simulink model "mVeh_fun_tbm"  (R2023b)
settings: Solver=FixedStepDiscrete  StartTime=0.0  StopTime=Parm_cnv_simulink_stopTime  FixedStep=Const_cnv_fundmt_stepSize  RelTol=1e-3  EnableMultiTasking=on
InitFcn:
  | preLoadFun
undefined symbols (not defined in the file or in its folder): Calib_pirelle_presSnr_x8, Calib_roadTriger_x6, Calib_tbm_brkBts_x8, Calib_tbm_ctr_x8, Calib_tbm_sensor_x4, Calib_tbm_strDistb_x8, Calib_tbm_supCtr_x8, CtrSet_tbm_enab_x8, IO397, Parm_tbmVeh_sig_max_numInvalid, Parm_tbmVeh_sig_tolerate_numInvalid
libraries: canmsglib x34, speedgoatlib_IO691 x19, MyLibrary x5, libtb_gen_canMsgCntr x5, speedgoatlib_fpga_analog_io x1, simulink x1, speedgoatlib_fpga x1, lib_decmp_CtrSet_tbm_enab_x8 x1, lib_decmp_Calib_tbm_brkPreTriger_x6 x1, lib_decmp_Calib_tbm_sensor_x4 x1
(part 1 of 3)
Description:
  | - Add preLoadFun.m into Callbacks InitFcn
  | - Combine Sensata and Pirelle sensor inputs into one subsystem
  | - Two enumerators: defEnum_fun_tbm.m && def_vehFun_Enum.m
settings Model: SimulationMode=external  PauseTimes=49.73  NumberOfSteps=20  PacingRate=112  Creator=jianjun.gao  LastModifiedBy=nolalala
settings SolverCC: ConcurrentTasks=on  AlgebraicLoopSolver=LineSearch  AutoInsertRateTranBlk=on
settings DataIOCC: LimitDataPoints=on  SaveFormat=StructureWithTime  ReturnWorkspaceOutputs=off
settings OptimizationCC: BlockReduction=off  DefaultUnderspecifiedDataType=single  OptimizeBlockIOStorage=off  EnhancedBackFolding=on  PassReuseOutputArgsThreshold=0  ExpressionDepthLimit=2147483647  OptimizeBlockOrder=speed  DifferentSizesBufferReuse=on
settings DebuggingCC: UnderspecifiedInitializationDetection=Classic  MergeDetectMultiDrivingBlocksExec=none  SolverPrmCheckMsg=warning  ParameterTunabilityLossMsg=error  FcnCallInpInsideContextMsg=warning  UnconnectedInputMsg=warning  UnconnectedOutputMsg=warning  UnconnectedLineMsg=warning  BusObjectLabelMismatch=error  AllowSymbolicDim=off  StateNameClashWarn=warning  SFUnexpectedBacktrackingDiag=warning  SFNoUnconditionalDefaultTransitionDiag=warning  SFExecutionAtInitializationDiag=none  ArithmeticOperatorsInVariantConditions=warning
settings HardwareCC: ProdBitPerPointer=32  ProdBitPerSizeT=32  ProdBitPerPtrDiffT=32  ProdLargestAtomicFloat=None  ProdWordSize=32  ProdLongLongMode=on  ProdHWDeviceType=Generic->32-bit x86 compatible
settings ModelReferenceCC: EnableRefExpFcnMdlSchedulingChecks=on  PropagateSignalLabelsOutOfModel=off
settings SFSimCC: SimUseLocalCustomCode=off  MATLABDynamicMemAlloc=off  CustomCodeUndefinedFunction=UseInterfaceOnly
settings RTWCC: Description=Simulink Real-Time  SystemTargetFile=slrt.tlc  PackageName=addn_compled  TemplateMakefile=slrt_default_tmf  RTWUseLocalCustomCode=off  RTWUseSimCustomCode=on  BuildConfiguration=Faster Runs  CodeExecutionProfiling=on  RTWCompilerOptimization=on
settings CodeAppCC: ForceParamTrailComments=on  MaxIdLength=63  OperatorAnnotations=on
settings SimulinkRealTimeCC: SupportVariableSizeSignals=on  OptimizeReductions=off  RL32LogTETModifier=off  xPCConcurrentTasks=on
settings ConfigComp: CovMetricSettings=dw  CovSaveCumulativeToWorkspaceVar=on  CovSaveSingleToWorkspaceVar=on  CovExternalEMLEnable=off
settings SimscapeCC: SimscapeNormalizeSystem=off
settings ConfigurationSet: Description=SimMechanics 2G

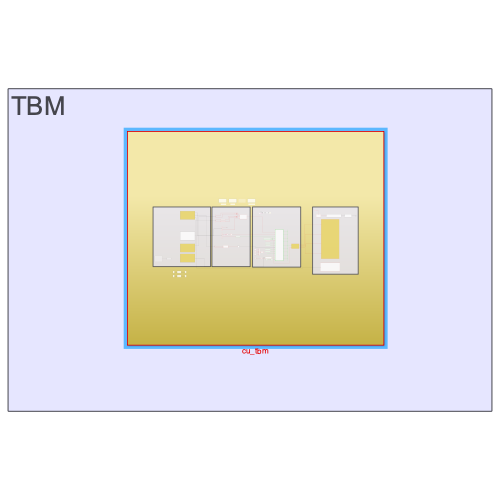
[thumbnail: Simulink's stored preview of the top-level diagram]
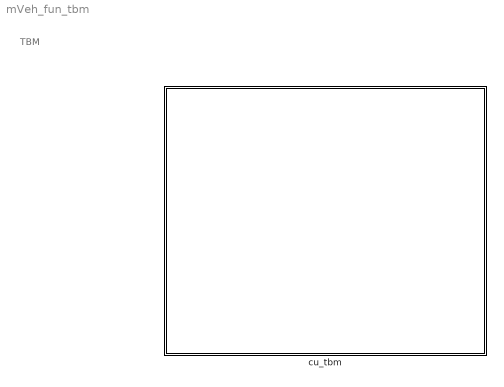
== system mVeh_fun_tbm ==
  note: TBM
  cu_tbm : Subsystem

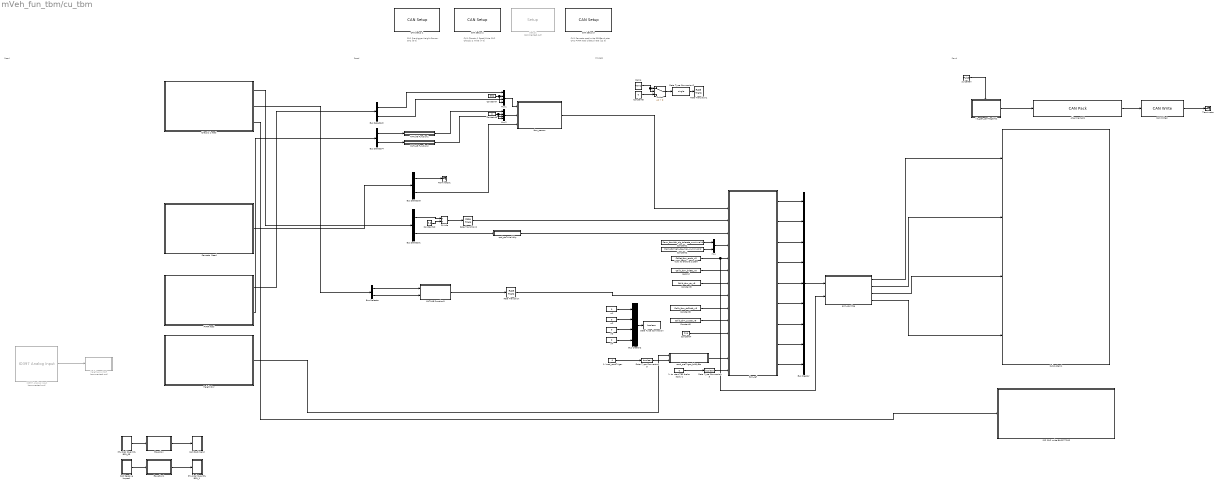
== system mVeh_fun_tbm/cu_tbm ==
  note: CH1 Pre-trigger Height Sensor
      | CH2
      | [6 0]
  note: Send
  note: Process
  note: Read
  note: CH1 Chassis 1 Read/Write
      | CH2 Chassis 2 Write
      | [7 0]
  note: CH1 Sensata read/write 500Baud rate
      | CH2 PVRR read 1kBaud rate
      | [12 0]
  note: Read
  1: load_roadTriger : Constant  Value=0  OutDataTypeStr=uint8  SampleTime=-1
  1: to  start TBS brake apply1 : Constant  Value=0  OutDataTypeStr=uint8  SampleTime=-1
  Alignment_01 : canmsglib/CAN Pack  CANdbFile=C:\Users\bowen.zheng\Desktop\spdGoat_prj_20230526_mod\spdGoat_prj_20230526\support\dbc\TBM_mix.dbc  MsgList=Alignment_01  MsgName=Alignment_01  MsgIDType=Standard (11-bit identifier)  MsgIdentifier=1043  MsgLength=2  Remote=off  ApplyMinMax=off  BusOutput=off  SignalInfo={'Alignment_TimeStamp','8','16','BE','unsigned','Standard','0','1','0','0','65535'}
      settings: DataFormat=CANdb specified signals
  Bus Creator : BusCreator  Inputs=9
  Bus Creator2 : BusCreator  Inputs=4
  Bus Selector : BusSelector  OutputSignals=BCU_04_BrkPedlTrvlCalSts,BCU_04_BrkPedlSts
  Bus Selector1 : BusSelector  OutputSignals=BCU_04_VehSpd,BCU_04_VehSpdSts
  Bus Selector2 : BusSelector  OutputSignals=PVRR_press_front,PVRR_press_rear
  Bus Selector3 : BusSelector  OutputSignals=Sensata_burst_pressure,Sensata_burst_flag
  Bus Selector4 : BusSelector  OutputSignals=PVRR_timestamp_front,PVRR_timestamp_rear
  CAN Pack Send : Subsystem
  CAN Receive Unpack : Subsystem
  CAN Setup 1 : speedgoatlib_IO691/CAN Setup   moduletype=IO691  id=1  pciSlot=[6 0]  chn1=CAN (HS)  chn2=CAN (HS)  chn3=Disabled  chn4=Disabled  initStruct=[]  termStruct=[]  ArbitrationbdrChn1=500 kBaud  ArbitrationManbdrChn1=[2,16,63,16]  FdbdrChn1=5.0 MBaud  FdManbdrChn1=[2,2,5,2]  ArbitrationbdrChn2=500 kBaud  ArbitrationManbdrChn2=[2,16,63,16]  FdbdrChn2=5.0 MBaud  FdManbdrChn2=[2,2,5,2]  ArbitrationbdrChn3=1.0 MBaud  ArbitrationManbdrChn3=[2,8,31,8]  FdbdrChn3=5.0 MBaud  FdManbdrChn3=[2,2,5,2]  ArbitrationbdrChn4=1.0 MBaud  ArbitrationManbdrChn4=[2,8,31,8]  FdbdrChn4=5.0 MBaud  FdManbdrChn4=[2,2,5,2]  moduleInitValues=[691 1 6 0]
  CAN Setup 2 : speedgoatlib_IO691/CAN Setup   moduletype=IO691  id=2  pciSlot=[7 0]  chn1=CAN (HS)  chn2=CAN (HS)  chn3=Disabled  chn4=Disabled  initStruct=[]  termStruct=[]  ArbitrationbdrChn1=500 kBaud  ArbitrationManbdrChn1=[2,16,63,16]  FdbdrChn1=5.0 MBaud  FdManbdrChn1=[2,2,5,2]  ArbitrationbdrChn2=500 kBaud  ArbitrationManbdrChn2=[2,16,63,16]  FdbdrChn2=5.0 MBaud  FdManbdrChn2=[2,2,5,2]  ArbitrationbdrChn3=1.0 MBaud  ArbitrationManbdrChn3=[2,8,31,8]  FdbdrChn3=5.0 MBaud  FdManbdrChn3=[2,2,5,2]  ArbitrationbdrChn4=1.0 MBaud  ArbitrationManbdrChn4=[2,8,31,8]  FdbdrChn4=5.0 MBaud  FdManbdrChn4=[2,2,5,2]  moduleInitValues=[691 2 7 0]
  CAN Setup 3 : speedgoatlib_IO691/CAN Setup   moduletype=IO691  id=4  pciSlot=[12 0]  chn1=CAN (HS)  chn2=CAN (HS)  chn3=Disabled  chn4=Disabled  initStruct=[]  termStruct=[]  ArbitrationbdrChn1=500 kBaud  ArbitrationManbdrChn1=[2,16,63,16]  FdbdrChn1=5.0 MBaud  FdManbdrChn1=[2,2,5,2]  ArbitrationbdrChn2=1.0 MBaud  ArbitrationManbdrChn2=[2,8,31,8]  FdbdrChn2=5.0 MBaud  FdManbdrChn2=[2,2,5,2]  ArbitrationbdrChn3=1.0 MBaud  ArbitrationManbdrChn3=[2,8,31,8]  FdbdrChn3=5.0 MBaud  FdManbdrChn3=[2,2,5,2]  ArbitrationbdrChn4=1.0 MBaud  ArbitrationManbdrChn4=[2,8,31,8]  FdbdrChn4=5.0 MBaud  FdManbdrChn4=[2,2,5,2]  moduleInitValues=[691 4 12 0]
  CAN Write2 : speedgoatlib_IO691/CAN Write  id=4  ts=0.01  channel=1  messageType=CAN  enableStatusPort=on  canType=CAN (HS)  initValues=[691 4 0.01 0 1 1 1]
  Chassis 1 read : Subsystem
  Constant1 : Constant  Value=Parm_tbmVeh_sig_tolerate_numInvalid  OutDataTypeStr=int8  SampleTime=-1
  Constant10 : Constant  Value=3.6  OutDataTypeStr=single
  Constant2 : Constant  Value=Parm_tbmVeh_sig_max_numInvalid  OutDataTypeStr=int8  SampleTime=-1
  Constant3 : Constant  Value=Calib_tbm_supCtr_x8  OutDataTypeStr=single  SampleTime=-1
  Constant4 : Constant  Value=true  OutDataTypeStr=boolean  SampleTime=-1
  Constant5 : Constant  Value=Calib_tbm_ctr_x8  OutDataTypeStr=single  SampleTime=-1
  Constant6 : Constant  Value=0  OutDataTypeStr=single
  Constant7 : Constant  Value=350  OutDataTypeStr=single  SampleTime=-1
  Constant8 : Constant  Value=Calib_tbm_strDistb_x8  OutDataTypeStr=single  SampleTime=-1
  Constant9 : Constant  Value=0  OutDataTypeStr=single  SampleTime=-1
  Data Type Conversion : DataTypeConversion  OutDataTypeStr=boolean  SaturateOnIntegerOverflow=off  RndMeth=Floor
  Data Type Conversion2 : DataTypeConversion  OutDataTypeStr=single  SaturateOnIntegerOverflow=off  RndMeth=Floor
  Data Type Conversion3 : DataTypeConversion  OutDataTypeStr=boolean  RndMeth=Nearest  SaturateOnIntegerOverflow=off
  Data Type Conversion5 : DataTypeConversion  OutDataTypeStr=boolean  RndMeth=Nearest  SaturateOnIntegerOverflow=off
  Divide : Product  Inputs=*/  OutDataTypeStr=single  RndMeth=Nearest
  Equation : Subsystem
  Equation1 : Subsystem
  Height Snr : Subsystem
  ID2 CH2 write BAICC TPMS : Subsystem
  IO397 Analog Input : speedgoatlib_fpga_analog_io/IO397 Analog Input  Commented=on  id=3  chan=[2:2]  range=+-10 V  trigger=Initiator  ts=0.001  pciSlot=-1  board=Please select...
  MATLAB Function1 : MATLAB Function  TreatAsAtomicUnit=on
  MATLAB Function2 : MATLAB Function  TreatAsAtomicUnit=on
  MATLAB Function3 : MATLAB Function  TreatAsAtomicUnit=on
  Mux : Mux  Inputs=2
  Mux1 : Mux
  Mux2 : Mux
  PVRR read : Subsystem
  Physical Quantity BCU_05 : Subsystem
  Physical Quantity BCU_1 : Subsystem
  Ramp : simulink/Sources/Ramp  slope=-2  start=10  InitialOutput=100
  Rate Transition : RateTransition
  Rate Transition1 : RateTransition
  Rate Transition2 : RateTransition
  Sensata  Read : Subsystem
  Setup1 : speedgoatlib_fpga/Setup/Setup  Commented=on  board=IO397-50k  id=3  device_id=1  frontIO=None  rearIO=None  bitstreamFile=speedgoat_IO397_50k_all_io.mat  rev=2.1  timestamp_string=06/12/19 11:07:30  fpgaFreq=75 MHz  fpgaTick=13.33 ns  ProgSpiFlash=off  ProgBPIFlash=off  pciSlot=-1  PullRPort0=pull-up 3.3V  VioPort0=3.3V  PullRPort1=pull-up 3.3V  VioPort1=3.3V  PullRPort2=pull-up 3.3V  VioPort2=3.3V  PullRPort3=pull-up 3.3V  VioPort3=3.3V  PullRPort4=pull-up 3.3V  VioPort4=3.3V  PullRPort5=pull-up 3.3V  VioPort5=3.3V  PullRPort6=pull-up 3.3V  VioPort6=3.3V  PullRPort15=pull-up 3.3V  PullRPort31=pull-up 3.3V  PullRPort47=pull-up 3.3V  PullRPort63=pull-up 3.3V
  Subsystem1 : Subsystem
  Switch : Switch  Criteria=u2 > Threshold  SaturateOnIntegerOverflow=off  InputSameDT=off
  Terminator : Terminator
  Terminator1 : Terminator
  asm_canMsg : Subsystem
  height_snr_VtoH : MATLAB Function  Commented=on  TreatAsAtomicUnit=on
  lib_gen_canMsgCntr1 : Stateflow chart  AncestorBlock=libtb_gen_canMsgCntr/lib_gen_canMsgCntr  TreatAsAtomicUnit=on
  pulseGen : DiscretePulseGenerator  PulseType=Time based  Period=0.01  PulseWidth=50
  road_preTriger_brkByBts : Subsystem
  second : Constant  Value=Calib_tbm_brkBts_x8  OutDataTypeStr=single  SampleTime=-1
  spd_stsToValidity : MATLAB Function  TreatAsAtomicUnit=on
  tbm_ref : ModelReference  ModelNameDialog=tbm_ref.slx  SimulationMode=Normal  ModelReferenceVersion=1.941
  tbm_sensor : Subsystem
  true: to enable system : Constant  Value=CtrSet_tbm_enab_x8  OutDataTypeStr=boolean  SampleTime=-1
  w1 : Constant  Value=0  OutDataTypeStr=single
  "w2 " : Constant  Value=0  OutDataTypeStr=single  SampleTime=-1
  w3 : Constant  Value=0  OutDataTypeStr=single  SampleTime=-1
  w4 : Constant  Value=0  OutDataTypeStr=single  SampleTime=-1
  wires:
  Chassis 1 read/2(BCU_04_BrkPedl_w_Sts) -> Bus Selector/1
  Chassis 1 read/1(BCU_04_VehSpd_w_Validity) -> Bus Selector1/1
  Sensata  Read/1(TPMS_TireBurst) -> Bus Selector3/1
  Chassis 1 read/3(BGW_02_VehState) -> ID2 CH2 write BAICC TPMS/1(VehState)
  Bus Creator2/1 -> Data Type Conversion/1
  "w2 "/1 -> Bus Creator2/2
  w1/1 -> Bus Creator2/1
  Bus Creator/1 -> asm_canMsg/1(cu_tbm)
  tbm_ref/1 -> Bus Creator/1  "tbm_st"
  tbm_ref/3 -> Bus Creator/3  "btsSimuDrBrk_mcp"
  tbm_ref/5 -> Bus Creator/5  "tbmModfBrk_pTgt_4w"
  tbm_ref/8 -> Bus Creator/8  "susp_ctrActv_4w"
  tbm_ref/2 -> Bus Creator/2  "btsSimuDrBrk_actv"
  tbm_ref/4 -> Bus Creator/4  "tbmModfBrk_actv_4w"
  spd_stsToValidity/1(spd_valid) -> tbm_ref/4
  tbm_ref/6 -> Bus Creator/6  "str_distbCtr_actv"
  tbm_ref/9 -> Bus Creator/9  "susp_pTgt_4w"
  tbm_ref/7 -> Bus Creator/7  "str_distbCtr_angTgt"
  Bus Selector3/1 -> Terminator1/1  "<Sensata_burst_pressure>"
  Bus Selector1/2 -> spd_stsToValidity/1(spd_status)  "<BCU_04_VehSpdSts>"
  Bus Selector/1 -> MATLAB Function3/1(brkPdlTrvlCalSts)  "<BCU_04_BrkPedlTrvlCalSts>"
  Bus Selector/2 -> MATLAB Function3/2(brkPdlSts)  "<BCU_04_BrkPedlSts>"
  Ramp/1 -> Switch/2, Switch/1
  asm_canMsg/4(bus_to_ch2_VCU_14) -> Subsystem1/4(busTo_vcu_14)
  asm_canMsg/3(busTo_adc1_eps_02) -> Subsystem1/3(busTo_adc1_eps_02)
  asm_canMsg/2(busTo_adc1_eps_01) -> Subsystem1/2(busTo_adc1_eps_01)
  asm_canMsg/1(busTo_ch1_tbm_02) -> Subsystem1/1(busTo_ch1_tbm_02)
  Constant6/1 -> Switch/3
  Switch/1 -> Data Type Conversion2/1
  Data Type Conversion2/1 -> Rate Transition1/1
  Bus Selector3/2 -> tbm_sensor/3(sansata_boutFlag_4w)  "<Sensata_burst_flag>"
  w3/1 -> Bus Creator2/3
  w4/1 -> Bus Creator2/4
  Bus Selector1/1 -> Divide/1  "<BCU_04_VehSpd>"
  Constant10/1 -> Divide/2
  Rate Transition2/1 -> tbm_ref/3
  Divide/1 -> Rate Transition2/1
  PVRR read/1(PVRR_press) -> Bus Selector2/1
  PVRR read/2(PVRR_timestamp) -> Bus Selector4/1
  Bus Selector2/1 -> Mux1/1  "<PVRR_press_front>"
  Bus Selector2/2 -> Mux1/3  "<PVRR_press_rear>"
  Bus Selector4/1 -> MATLAB Function1/1(timestamp)  "<PVRR_timestamp_front>"
  Bus Selector4/2 -> MATLAB Function2/1(timestamp)  "<PVRR_timestamp_rear>"
  IO397 Analog Input/1 -> height_snr_VtoH/1(snr_volt)  "Analog Input"
  pulseGen/1 -> lib_gen_canMsgCntr1/Trigger
  Alignment_01/1 -> CAN Write2/1
  lib_gen_canMsgCntr1/1(count) -> Alignment_01/1  "Alightment_cout"
  CAN Write2/1 -> Terminator/1  "state"
  1: to  start TBS brake apply1/1 -> Data Type Conversion3/1  "handTriger"
  Data Type Conversion3/1 -> tbm_ref/15
  Data Type Conversion5/1 -> road_preTriger_brkByBts/2(load_roadTrigr)
  road_preTriger_brkByBts/1(road_trigred) -> tbm_ref/14  "road_trigred"
  1: load_roadTriger/1 -> Data Type Conversion5/1  "load_roadTriger"
  Constant4/1 -> tbm_ref/12
  Constant3/1 -> tbm_ref/11
  Constant8/1 -> tbm_ref/10
  MATLAB Function3/1(dr_isBrkg) -> Rate Transition/1  "dr_isBrkg"
  Constant5/1 -> tbm_ref/8
  second/1 -> tbm_ref/7
  true: to enable system/1 -> tbm_ref/6, asm_canMsg/2(CtrSet_tbm_enab_x8)
  Mux/1 -> tbm_ref/5
  Constant1/1 -> Mux/1
  Constant2/1 -> Mux/2
  Height Snr/1(Height Snr) -> road_preTriger_brkByBts/1(measured_tgrGap)  "height_snr"
  Rate Transition/1 -> tbm_ref/9
  Constant9/1 -> Mux2/4, Mux2/2
  Constant7/1 -> Mux1/2, Mux1/4
  Mux1/1 -> tbm_sensor/1(pirelle_tryPres_4w)
  Mux2/1 -> tbm_sensor/2(pirelle_snrTime_4w)
  tbm_sensor/1(snr_boutFlag_4w) -> tbm_ref/2  "snr_blouFlag_4w"
  MATLAB Function1/1(timestamp_sec) -> Mux2/1  "ts_sec_front"
  MATLAB Function2/1(timestamp_sec) -> Mux2/3  "ts_sec_rear"
  Physical Quantity BCU_05/1(BCU_05) -> Equation/1(BCU_05)
  Equation/1(Transformed) -> CAN Pack Send/1(Input)
  CAN Receive Unpack/1(Output) -> Equation1/1(ADC_Waypoint)
  Equation1/1(Transformed) -> Physical Quantity BCU_1/1(Input)

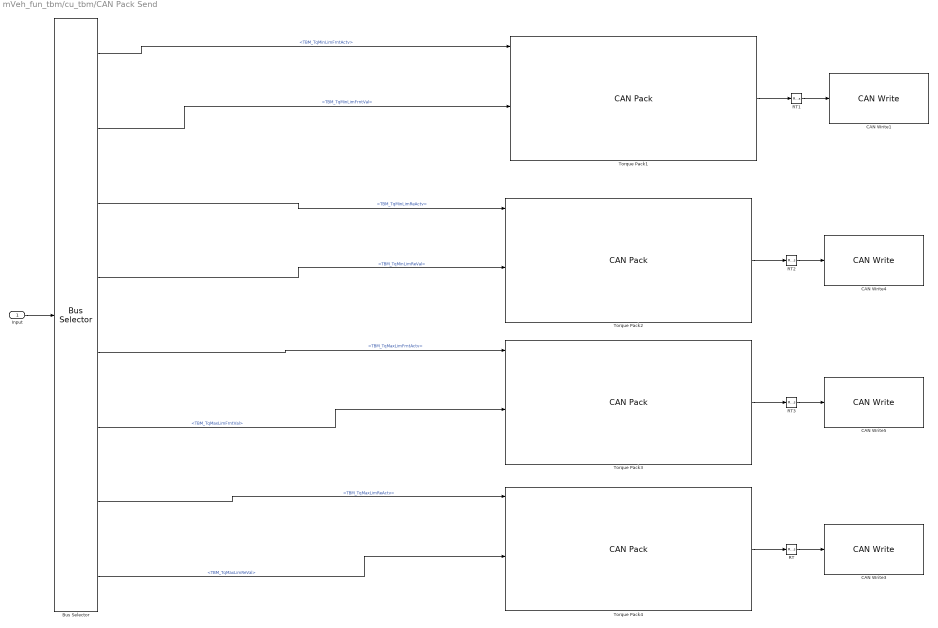
== system mVeh_fun_tbm/cu_tbm/CAN Pack Send ==
  Input : Inport
  Bus Selector : BusSelector  OutputSignals=TBM_TqMinLimFrntActv,TBM_TqMinLimFrntVal,TBM_TqMinLimReActv,TBM_TqMinLimReVal,TBM_TqMaxLimFrntActv,TBM_TqMaxLimFrntVal,TBM_TqMaxLimReActv,TBM_TqMaxLimReVal
  CAN Write{1,3..5} (4 alike) : speedgoatlib_IO691/CAN Write  id=2  ts=0.02  channel=1  messageType=CAN  enableStatusPort=off  canType=CAN (HS)  initValues=[691 2 0.02 0 1 1 0]
  RT{,1..3} (4 alike) : RateTransition  OutPortSampleTime=0.02
  Torque Pack1 : canmsglib/CAN Pack  CANdbFile=.\support\dbc\NIO_NT2_Chassis2_CAN_Official_Release_V_1_1_DA_02.dbc  MsgList=ADC1_WayPoint01  MsgName=ADC1_WayPoint01  MsgIDType=Standard (11-bit identifier)  MsgIdentifier=214  MsgLength=8  Remote=off  ApplyMinMax=off  BusOutput=off  SignalInfo={'LD_Confidence_1','24','4','BE','unsigned','Standard','0','0.1','0','0','1.5';'LD_First_End_1','51','7','BE','unsigned','Standard','0','1','0','0','127';'LD_First_Start_1','16','8','BE','unsigned','Standard','0','0.1','0','0','25.5';'LD_First_Type_1','28','4','BE','unsigned','Standard','0','1','0','0','15';'LD_Line_First_C0_1','56','11','BE','unsigned','Standard','0','0.01','-10.24','-10.24','10.23';'LD_Line_First_C1_1','43','13','BE','unsigned','Standard','0','0.0001','-0.4096','-0.4096','0.4095';'LD_Line_First_C2_1','0','8','BE','unsigned','Standard','0','0.0001','-0.0128','-0.0128','0.0127';'LD_Line_First_C3_1','8','8','BE','unsigned','Standard','0','1e-06','-0.000128','-0.000128','0.000127'}
      settings: DataFormat=CANdb specified signals
  Torque Pack2 : canmsglib/CAN Pack  CANdbFile=.\support\dbc\NIO_NT2_Chassis2_CAN_Official_Release_V_1_1_DA_02.dbc  MsgList=ADC1_WayPoint02  MsgName=ADC1_WayPoint02  MsgIDType=Standard (11-bit identifier)  MsgIdentifier=215  MsgLength=8  Remote=off  ApplyMinMax=off  BusOutput=off  SignalInfo={'LD_Confidence_2','24','4','BE','unsigned','Standard','0','0.1','0','0','1.5';'LD_First_End_2','51','7','BE','unsigned','Standard','0','1','0','0','127';'LD_First_Start_2','16','8','BE','unsigned','Standard','0','0.1','0','0','25.5';'LD_First_Type_2','28','4','BE','unsigned','Standard','0','1','0','0','15';'LD_Line_First_C0_2','56','11','BE','unsigned','Standard','0','0.01','-10.24','-10.24','10.23';'LD_Line_First_C1_2','43','13','BE','unsigned','Standard','0','0.0001','-0.4096','-0.4096','0.4095';'LD_Line_First_C2_2','0','8','BE','unsigned','Standard','0','0.0001','-0.0128','-0.0128','0.0127';'LD_Line_First_C3_2','8','8','BE','unsigned','Standard','0','1e-06','-0.000128','-0.000128','0.000127'}
      settings: DataFormat=CANdb specified signals
  Torque Pack3 : canmsglib/CAN Pack  CANdbFile=.\support\dbc\NIO_NT2_Chassis2_CAN_Official_Release_V_1_1_DA_02.dbc  MsgList=ADC1_WayPoint03  MsgName=ADC1_WayPoint03  MsgIDType=Standard (11-bit identifier)  MsgIdentifier=216  MsgLength=8  Remote=off  ApplyMinMax=off  BusOutput=off  SignalInfo={'LD_Confidence_3','24','4','BE','unsigned','Standard','0','0.1','0','0','1.5';'LD_First_End_3','51','7','BE','unsigned','Standard','0','1','0','0','127';'LD_First_Start_3','16','8','BE','unsigned','Standard','0','0.1','0','0','25.5';'LD_First_Type_3','28','4','BE','unsigned','Standard','0','1','0','0','15';'LD_Line_First_C0_3','56','11','BE','unsigned','Standard','0','0.01','-10.24','-10.24','10.23';'LD_Line_First_C1_3','43','13','BE','unsigned','Standard','0','0.0001','-0.4096','-0.4096','0.4095';'LD_Line_First_C2_3','0','8','BE','unsigned','Standard','0','0.0001','-0.0128','-0.0128','0.0127';'LD_Line_First_C3_3','8','8','BE','unsigned','Standard','0','1e-06','-0.000128','-0.000128','0.000127'}
      settings: DataFormat=CANdb specified signals
  Torque Pack4 : canmsglib/CAN Pack  CANdbFile=.\support\dbc\NIO_NT2_Chassis2_CAN_Official_Release_V_1_1_DA_02.dbc  MsgList=ADC1_WayPoint04  MsgName=ADC1_WayPoint04  MsgIDType=Standard (11-bit identifier)  MsgIdentifier=217  MsgLength=8  Remote=off  ApplyMinMax=off  BusOutput=off  SignalInfo={'LD_Confidence_4','24','4','BE','unsigned','Standard','0','0.1','0','0','1.5';'LD_First_End_4','51','7','BE','unsigned','Standard','0','1','0','0','127';'LD_First_Start_4','16','8','BE','unsigned','Standard','0','0.1','0','0','25.5';'LD_First_Type_4','28','4','BE','unsigned','Standard','0','1','0','0','15';'LD_Line_First_C0_4','56','11','BE','unsigned','Standard','0','0.01','-10.24','-10.24','10.23';'LD_Line_First_C1_4','43','13','BE','unsigned','Standard','0','0.0001','-0.4096','-0.4096','0.4095';'LD_Line_First_C2_4','0','8','BE','unsigned','Standard','0','0.0001','-0.0128','-0.0128','0.0127';'LD_Line_First_C3_4','8','8','BE','unsigned','Standard','0','1e-06','-0.000128','-0.000128','0.000127'}
      settings: DataFormat=CANdb specified signals
  wires:
  RT/1 -> CAN Write3/1
  RT3/1 -> CAN Write5/1
  Torque Pack3/1 -> RT3/1
  Torque Pack4/1 -> RT/1
  Torque Pack2/1 -> RT2/1
  RT2/1 -> CAN Write4/1
  Input/1 -> Bus Selector/1
  Bus Selector/1 -> Torque Pack1/1  "<TBM_TqMinLimFrntActv>"
  RT1/1 -> CAN Write1/1
  Torque Pack1/1 -> RT1/1
  Bus Selector/2 -> Torque Pack1/5  "<TBM_TqMinLimFrntVal>"
  Bus Selector/3 -> Torque Pack2/1  "<TBM_TqMinLimReActv>"
  Bus Selector/4 -> Torque Pack2/5  "<TBM_TqMinLimReVal>"
  Bus Selector/5 -> Torque Pack3/1  "<TBM_TqMaxLimFrntActv>"
  Bus Selector/6 -> Torque Pack3/5  "<TBM_TqMaxLimFrntVal>"
  Bus Selector/7 -> Torque Pack4/1  "<TBM_TqMaxLimReActv>"
  Bus Selector/8 -> Torque Pack4/5  "<TBM_TqMaxLimReVal>"

== system mVeh_fun_tbm/cu_tbm/CAN Receive Unpack ==
  CAN Read2 : speedgoatlib_IO691/CAN Read  id=2  ts=-1  channel=1  messageType=CAN  canType=CAN (HS)  initValues=[691 2 -1 0 1 1]
  Subsystem : Subsystem
  While Iterator : WhileIterator  MaxIters=-1  WhileBlockType=do-while
  Output : Outport
  wires:
  CAN Read2/2 -> Subsystem/1(In1)
  CAN Read2/1 -> While Iterator/1
  Subsystem/1(Output) -> Output/1

== system mVeh_fun_tbm/cu_tbm/Chassis 1 read ==
  CAN Read2 : speedgoatlib_IO691/CAN Read  id=2  ts=-1  channel=1  messageType=CAN  canType=CAN (HS)  initValues=[691 2 -1 0 1 1]
  Subsystem : Subsystem
  While Iterator : WhileIterator  MaxIters=-1  WhileBlockType=do-while
  BCU_04_VehSpd_w_Validity : Outport
  BCU_04_BrkPedl_w_Sts : Outport  Port=2
  BGW_02_VehState : Outport  Port=3
  wires:
  CAN Read2/1 -> While Iterator/1
  CAN Read2/2 -> Subsystem/1(In1)
  Subsystem/2(BCU_04_BrkPedl_w_Sts) -> BCU_04_BrkPedl_w_Sts/1
  Subsystem/1(BCU_04_VehSpd_w_Validity) -> BCU_04_VehSpd_w_Validity/1
  Subsystem/3(BGW_02_VehState) -> BGW_02_VehState/1

== system mVeh_fun_tbm/cu_tbm/Equation ==
  BCU_05 : Inport
  Bus Creator : BusCreator  Inputs=8
  Bus Selector : BusSelector  OutputSignals=TBM_TqMinLimFrntActv,TBM_TqMinLimFrntVal,TBM_TqMinLimReActv,TBM_TqMinLimReVal,TBM_TqMaxLimFrntActv,TBM_TqMaxLimFrntVal,TBM_TqMaxLimReActv,TBM_TqMaxLimReVal
  MATLAB Function : MATLAB Function  TreatAsAtomicUnit=on
  MATLAB Function1 : MATLAB Function  TreatAsAtomicUnit=on
  MATLAB Function2 : MATLAB Function  TreatAsAtomicUnit=on
  MATLAB Function3 : MATLAB Function  TreatAsAtomicUnit=on
  Transformed : Outport
  wires:
  BCU_05/1 -> Bus Selector/1
  Bus Creator/1 -> Transformed/1
  Bus Selector/1 -> Bus Creator/1  "<TBM_TqMinLimFrntActv>"
  Bus Selector/3 -> Bus Creator/3  "<TBM_TqMinLimReActv>"
  Bus Selector/5 -> Bus Creator/5  "<TBM_TqMaxLimFrntActv>"
  Bus Selector/7 -> Bus Creator/7  "<TBM_TqMaxLimReActv>"
  Bus Selector/2 -> MATLAB Function/1(u)  "<TBM_TqMinLimFrntVal>"
  MATLAB Function/1(y) -> Bus Creator/2  "TBM_TqMinLimFrntVal"
  Bus Selector/8 -> MATLAB Function3/1(u)  "<TBM_TqMaxLimReVal>"
  Bus Selector/6 -> MATLAB Function2/1(u)  "<TBM_TqMaxLimFrntVal>"
  Bus Selector/4 -> MATLAB Function1/1(u)  "<TBM_TqMinLimReVal>"
  MATLAB Function1/1(y) -> Bus Creator/4  "TBM_TqMinLimReVal"
  MATLAB Function2/1(y) -> Bus Creator/6  "TBM_TqMaxLimFrntVal"
  MATLAB Function3/1(y) -> Bus Creator/8  "TBM_TqMaxLimReVal"

== system mVeh_fun_tbm/cu_tbm/Equation1 ==
  ADC_Waypoint : Inport
  Bus Creator : BusCreator  Inputs=8
  Bus Selector : BusSelector  OutputSignals=TBM_TqMinLimFrntActv,LD_Line_First_C0_1,TBM_TqMinLimReActv,LD_Line_First_C0_2,TBM_TqMaxLimFrntActv,LD_Line_First_C0_3,TBM_TqMaxLimReActv,LD_Line_First_C0_4
  MATLAB Function : MATLAB Function  TreatAsAtomicUnit=on
  MATLAB Function1 : MATLAB Function  TreatAsAtomicUnit=on
  MATLAB Function2 : MATLAB Function  TreatAsAtomicUnit=on
  MATLAB Function3 : MATLAB Function  TreatAsAtomicUnit=on
  Transformed : Outport
  wires:
  ADC_Waypoint/1 -> Bus Selector/1
  Bus Creator/1 -> Transformed/1
  Bus Selector/1 -> Bus Creator/1  "<TBM_TqMinLimFrntActv>"
  Bus Selector/3 -> Bus Creator/3  "<TBM_TqMinLimReActv>"
  Bus Selector/5 -> Bus Creator/5  "<TBM_TqMaxLimFrntActv>"
  Bus Selector/7 -> Bus Creator/7  "<TBM_TqMaxLimReActv>"
  Bus Selector/2 -> MATLAB Function/1(u)  "<LD_Line_First_C0_1>"
  MATLAB Function/1(y) -> Bus Creator/2  "TBM_TqMinLimFrntVal"
  Bus Selector/8 -> MATLAB Function3/1(u)  "<LD_Line_First_C0_4>"
  Bus Selector/6 -> MATLAB Function2/1(u)  "<LD_Line_First_C0_3>"
  Bus Selector/4 -> MATLAB Function1/1(u)  "<LD_Line_First_C0_2>"
  MATLAB Function1/1(y) -> Bus Creator/4  "TBM_TqMinLimReVal"
  MATLAB Function2/1(y) -> Bus Creator/6  "TBM_TqMaxLimFrntVal"
  MATLAB Function3/1(y) -> Bus Creator/8  "TBM_TqMaxLimReVal"

== system mVeh_fun_tbm/cu_tbm/Height Snr ==
  CAN Read2 : speedgoatlib_IO691/CAN Read  id=1  ts=-1  channel=1  messageType=CAN  canType=CAN (HS)  initValues=[691 1 -1 0 1 1]
  Subsystem : Subsystem
  While Iterator : WhileIterator  MaxIters=-1  WhileBlockType=do-while
  Height Snr : Outport
  wires:
  CAN Read2/1 -> While Iterator/1
  CAN Read2/2 -> Subsystem/1(In1)
  Subsystem/1(Height) -> Height Snr/1

== system mVeh_fun_tbm/cu_tbm/ID2 CH2 write BAICC TPMS ==
  VehState : Inport
  CAN Write2 : speedgoatlib_IO691/CAN Write  id=4  ts=0.1  channel=1  messageType=CAN  enableStatusPort=off  canType=CAN (HS)  initValues=[691 4 0.1 0 1 1 0]
  CM3 : canmsglib/CAN Pack  CANdbFile=D:\Desktop\spdGoat_prj_20230526\spdGoat_prj_20230526\support\dbc\BAICC_HC1_TPMS_Matrix_J1939_V1.0.dbc  MsgList=(none)  MsgName=CM3  MsgIDType=Extended (29-bit identifier)  MsgIdentifier=419288097  MsgLength=8  Remote=off  ApplyMinMax=off  BusOutput=off  SignalInfo={'KeySwitchIgnitionPower','20','2','LE','unsigned','Standard','0','1','0','0','3'}
      settings: DataFormat=CANdb specified signals
  Data Type Conversion : DataTypeConversion  OutDataTypeStr=boolean  SaturateOnIntegerOverflow=off  RndMeth=Floor
  wires:
  CM3/1 -> CAN Write2/1
  Data Type Conversion/1 -> CM3/1
  VehState/1 -> Data Type Conversion/1

== system mVeh_fun_tbm/cu_tbm/PVRR read ==
  CAN Read2 : speedgoatlib_IO691/CAN Read  id=4  ts=-1  channel=2  messageType=CAN  canType=CAN (HS)  initValues=[691 4 -1 1 1 1]
  Subsystem : Subsystem
  While Iterator : WhileIterator  MaxIters=-1  WhileBlockType=do-while
  PVRR_press : Outport
  PVRR_timestamp : Outport  Port=2
  wires:
  CAN Read2/1 -> While Iterator/1
  CAN Read2/2 -> Subsystem/1(In1)
  Subsystem/1(PVRR_press) -> PVRR_press/1
  Subsystem/2(PVRR_timestamp) -> PVRR_timestamp/1

== system mVeh_fun_tbm/cu_tbm/Physical Quantity BCU_05 ==
  Bus Creator1 : BusCreator  Inputs=8
  TBM_TqMaxLimFrntActv : Constant  OutDataTypeStr=single
  TBM_TqMaxLimFrntVal : Constant  OutDataTypeStr=single
  TBM_TqMaxLimReActv : Constant  OutDataTypeStr=single
  TBM_TqMaxLimReVal : Constant  OutDataTypeStr=single
  TBM_TqMinLimFrntActv : Constant  OutDataTypeStr=single
  TBM_TqMinLimFrntVal : Constant  OutDataTypeStr=single
  TBM_TqMinLimReActv : Constant  OutDataTypeStr=single
  TBM_TqMinLimReVal : Constant  OutDataTypeStr=single
  BCU_05 : Outport  OutDataTypeStr=single  PortDimensions=8
  wires:
  TBM_TqMaxLimReVal/1 -> Bus Creator1/8  "TBM_TqMaxLimReVal"
  Bus Creator1/1 -> BCU_05/1
  TBM_TqMinLimFrntVal/1 -> Bus Creator1/2  "TBM_TqMinLimFrntVal"
  TBM_TqMinLimReVal/1 -> Bus Creator1/4  "TBM_TqMinLimReVal"
  TBM_TqMinLimReActv/1 -> Bus Creator1/3  "TBM_TqMinLimReActv"
  TBM_TqMaxLimFrntActv/1 -> Bus Creator1/5  "TBM_TqMaxLimFrntActv"
  TBM_TqMaxLimReActv/1 -> Bus Creator1/7  "TBM_TqMaxLimReActv"
  TBM_TqMinLimFrntActv/1 -> Bus Creator1/1  "TBM_TqMinLimFrntActv"
  TBM_TqMaxLimFrntVal/1 -> Bus Creator1/6  "TBM_TqMaxLimFrntVal"

== system mVeh_fun_tbm/cu_tbm/Physical Quantity BCU_1 ==
  Input : Inport
  Bus Selector : BusSelector  OutputSignals=TBM_TqMinLimFrntActv,TBM_TqMinLimFrntVal,TBM_TqMinLimReActv,TBM_TqMinLimReVal,TBM_TqMaxLimFrntActv,TBM_TqMaxLimFrntVal,TBM_TqMaxLimReActv,TBM_TqMaxLimReVal
  wires:
  Bus Selector/8 -> ?  "<TBM_TqMaxLimReVal>"
  Bus Selector/2 -> ?  "<TBM_TqMinLimFrntVal>"
  Bus Selector/4 -> ?  "<TBM_TqMinLimReVal>"
  Bus Selector/3 -> ?  "<TBM_TqMinLimReActv>"
  Bus Selector/5 -> ?  "<TBM_TqMaxLimFrntActv>"
  Bus Selector/7 -> ?  "<TBM_TqMaxLimReActv>"
  Bus Selector/1 -> ?  "<TBM_TqMinLimFrntActv>"
  Bus Selector/6 -> ?  "<TBM_TqMaxLimFrntVal>"
  Input/1 -> Bus Selector/1

== system mVeh_fun_tbm/cu_tbm/Sensata  Read ==
  CAN Read2 : speedgoatlib_IO691/CAN Read  id=4  ts=-1  channel=1  messageType=CAN  canType=CAN (HS)  initValues=[691 4 -1 0 1 1]
  Subsystem : Subsystem
  While Iterator : WhileIterator  MaxIters=-1  WhileBlockType=do-while
  TPMS_TireBurst : Outport
  wires:
  CAN Read2/1 -> While Iterator/1
  CAN Read2/2 -> Subsystem/1(In1)
  Subsystem/1(TPMS_TireBurst) -> TPMS_TireBurst/1

== system mVeh_fun_tbm/cu_tbm/Subsystem1 ==
  busTo_ch1_tbm_02 : Inport  PortDimensions=10
  busTo_adc1_eps_01 : Inport  Port=2
  busTo_adc1_eps_02 : Inport  Port=3
  busTo_vcu_14 : Inport  Port=4
  " write TBM_02" : Subsystem
  send_ADC1_EPS_1AND2 : Subsystem
  write BCU_09 : Subsystem
  write VCU_14 : Subsystem
  wires:
  busTo_vcu_14/1 -> write VCU_14/1(cmd_brk_4whPres)
  busTo_ch1_tbm_02/1 -> " write TBM_02"/1(Input)
  busTo_adc1_eps_01/1 -> send_ADC1_EPS_1AND2/1(busTo_adc1_eps)
  busTo_adc1_eps_02/1 -> send_ADC1_EPS_1AND2/2(busTo_adc1_eps_02)

== system mVeh_fun_tbm/cu_tbm/asm_canMsg ==
  cu_tbm : Inport
  CtrSet_tbm_enab_x8 : Inport  Port=2  OutDataTypeStr=boolean  PortDimensions=8
  Bus Selector : BusSelector  OutputSignals=enable_TBM_suspCtr,enable_EPS_distb,enable_BTS_simuDrBrk
  lib_decmp_CtrSet_tbm_enab_x8 : lib_decmp_CtrSet_tbm_enab_x8/lib_decmp_CtrSet_tbm_enab_x8  SystemSampleTime=-1  VariantActivationTime=update diagram  AllowFlexibleInterface=on  Latency=0  AutoFrameSizeCalculation=off
  to_bcu_bts : Subsystem
  to_eps : Subsystem
  to_suspension : Subsystem
  busTo_ch1_tbm_02 : Outport
  busTo_adc1_eps_01 : Outport  Port=2
  busTo_adc1_eps_02 : Outport  Port=3
  bus_to_ch2_VCU_14 : Outport  Port=4
  wires:
  cu_tbm/1 -> to_bcu_bts/2(cu_tbm), to_eps/2(cu_tbm), to_suspension/2(cu_tbm)
  CtrSet_tbm_enab_x8/1 -> lib_decmp_CtrSet_tbm_enab_x8/1
  lib_decmp_CtrSet_tbm_enab_x8/1 -> Bus Selector/1
  Bus Selector/1 -> to_suspension/1(suspCtr_enab)  "<enable_TBM_suspCtr>"
  Bus Selector/2 -> to_eps/1(epsDist_enab)  "<enable_EPS_distb>"
  Bus Selector/3 -> to_bcu_bts/1(bts_enab)  "<enable_BTS_simuDrBrk>"
  to_suspension/1(busTo_ch1_tbm_02) -> busTo_ch1_tbm_02/1
  to_eps/2(busTo_adc1_eps_02) -> busTo_adc1_eps_02/1
  to_eps/1(busTo_adc1_eps_01) -> busTo_adc1_eps_01/1
  to_bcu_bts/1(bus_to_ch2_VCU_14) -> bus_to_ch2_VCU_14/1

== system mVeh_fun_tbm/cu_tbm/road_preTriger_brkByBts ==
  measured_tgrGap : Inport  OutDataTypeStr=double
  load_roadTrigr : Inport  Port=2  OutDataTypeStr=boolean
  Bus Selector1 : BusSelector  OutputSignals=gapMax,gapMin,numDatMin
  Constant11 : Constant  Value=Calib_roadTriger_x6  OutDataTypeStr=single  SampleTime=-1
  Data Type Conversion : DataTypeConversion  OutDataTypeStr=single  SaturateOnIntegerOverflow=off  RndMeth=Floor
  MATLAB Function : MATLAB Function  TreatAsAtomicUnit=on
  Terminator : Terminator
  Terminator1 : Terminator
  Unit Delay : UnitDelay  SampleTime=-1  HasFrameUpgradeWarning=on
  lib_decmp_Calib_tbm_brkPreTriger_x6 : lib_decmp_Calib_tbm_brkPreTriger_x6/lib_decmp_Calib_tbm_brkPreTriger_x6  SystemSampleTime=-1  VariantActivationTime=update diagram  AllowFlexibleInterface=on  Latency=0  AutoFrameSizeCalculation=off
  sm_trigr_byHeitSnr : Stateflow chart  TreatAsAtomicUnit=on
  road_trigred : Outport
  wires:
  Bus Selector1/2 -> sm_trigr_byHeitSnr/5(clb_gapMin)  "<gapMin>"
  Bus Selector1/1 -> sm_trigr_byHeitSnr/4(clb_gapMax)  "<gapMax>"
  Unit Delay/1 -> MATLAB Function/1(old_measure)
  MATLAB Function/1(measure_isNew) -> sm_trigr_byHeitSnr/1(measure_isNew)  "measure_isNew"
  measured_tgrGap/1 -> Unit Delay/1, MATLAB Function/2(new_measure), Data Type Conversion/1
  load_roadTrigr/1 -> sm_trigr_byHeitSnr/3(load_trigr)
  sm_trigr_byHeitSnr/1(trigred) -> road_trigred/1
  Constant11/1 -> lib_decmp_Calib_tbm_brkPreTriger_x6/1
  lib_decmp_Calib_tbm_brkPreTriger_x6/1 -> Bus Selector1/1
  Bus Selector1/3 -> sm_trigr_byHeitSnr/6(clb_numDatMin)  "<numDatMin>"
  Data Type Conversion/1 -> sm_trigr_byHeitSnr/2(measured_tgrGap)
  sm_trigr_byHeitSnr/2(st) -> Terminator/1  "st_sm_trigr_byHeitSnr"
  sm_trigr_byHeitSnr/3(qalfd_numDat) -> Terminator1/1  "qalfd_numDat"

== system mVeh_fun_tbm/cu_tbm/tbm_sensor ==
  pirelle_tryPres_4w : Inport  OutDataTypeStr=single  PortDimensions=4
  pirelle_snrTime_4w : Inport  Port=2  OutDataTypeStr=single  PortDimensions=4
  sansata_boutFlag_4w : Inport  Port=3  OutDataTypeStr=boolean  PortDimensions=4
  Bus Selector2 : BusSelector  OutputSignals=tbmSnr_type,tbmSnr_timeDelay
  Constant11 : Constant  Value=Calib_tbm_sensor_x4  SampleTime=-1
  Constant6 : Constant  Value=Calib_pirelle_presSnr_x8  OutDataTypeStr=single  SampleTime=-1
  lib_decmp_Calib_tbm_sensor_x4 : lib_decmp_Calib_tbm_sensor_x4/lib_decmp_Calib_tbm_sensor_x4  SystemSampleTime=-1  VariantActivationTime=update diagram  AllowFlexibleInterface=on  Latency=0  AutoFrameSizeCalculation=off
  perSnrType_enab : MATLAB Function  TreatAsAtomicUnit=on
  perSnrType_selectOut : MATLAB Function  TreatAsAtomicUnit=on
  tbm_pirelleSnr_ref : ModelReference  ModelNameDialog=tbm_pirelleSnr_ref.slx  SimulationMode=Normal  ModelReferenceVersion=1.851  EnablePortName=Enable  EnablePortStatesWhenEnabling=held
  snr_boutFlag_4w : Outport  OutDataTypeStr=boolean  PortDimensions=4
  wires:
  Bus Selector2/2 -> tbm_pirelleSnr_ref/4  "<tbmSnr_timeDelay>"
  pirelle_snrTime_4w/1 -> tbm_pirelleSnr_ref/2
  sansata_boutFlag_4w/1 -> perSnrType_selectOut/3(sansata_boutFlag_4w)
  tbm_pirelleSnr_ref/1 -> perSnrType_selectOut/2(pirelle_boutFlag_4w)  "pirelle_flag"
  perSnrType_selectOut/1(boutFlag_4w) -> snr_boutFlag_4w/1
  perSnrType_enab/1(enab_Pirelle) -> tbm_pirelleSnr_ref/Enable  "enab_Pirelli"
  Bus Selector2/1 -> perSnrType_enab/1(snrType), perSnrType_selectOut/1(snrType)  "<tbmSnr_type>"
  Constant6/1 -> tbm_pirelleSnr_ref/3
  Constant11/1 -> lib_decmp_Calib_tbm_sensor_x4/1
  pirelle_tryPres_4w/1 -> tbm_pirelleSnr_ref/1
  lib_decmp_Calib_tbm_sensor_x4/1 -> Bus Selector2/1
  perSnrType_enab/2(enab_Sansata) -> ?

== system mVeh_fun_tbm/cu_tbm/CAN Receive Unpack/Subsystem ==
  In1 : Inport
  ADC_Waypoint1 : Subsystem
  ADC_Waypoint2 : Subsystem
  ADC_Waypoint3 : Subsystem
  ADC_Waypoint4 : Subsystem
  Bus Creator : BusCreator  Inputs=8
  Output : Outport
  wires:
  In1/1 -> ADC_Waypoint4/1(In1), ADC_Waypoint3/1(In1), ADC_Waypoint2/1(In1), ADC_Waypoint1/1(In1)
  ADC_Waypoint1/1(LD_Confidence_1) -> Bus Creator/1  "TBM_TqMinLimFrntActv"
  ADC_Waypoint1/2(LD_Line_First_C0_1) -> Bus Creator/2
  ADC_Waypoint2/1(LD_Confidence_2) -> Bus Creator/3  "TBM_TqMinLimReActv"
  ADC_Waypoint2/2(LD_Line_First_C0_2) -> Bus Creator/4
  ADC_Waypoint3/1(LD_Confidence_3) -> Bus Creator/5  "TBM_TqMaxLimFrntActv"
  ADC_Waypoint3/2(LD_Line_First_C0_3) -> Bus Creator/6
  ADC_Waypoint4/1(LD_Confidence_4) -> Bus Creator/7  "TBM_TqMaxLimReActv"
  ADC_Waypoint4/2(LD_Line_First_C0_4) -> Bus Creator/8
  Bus Creator/1 -> Output/1

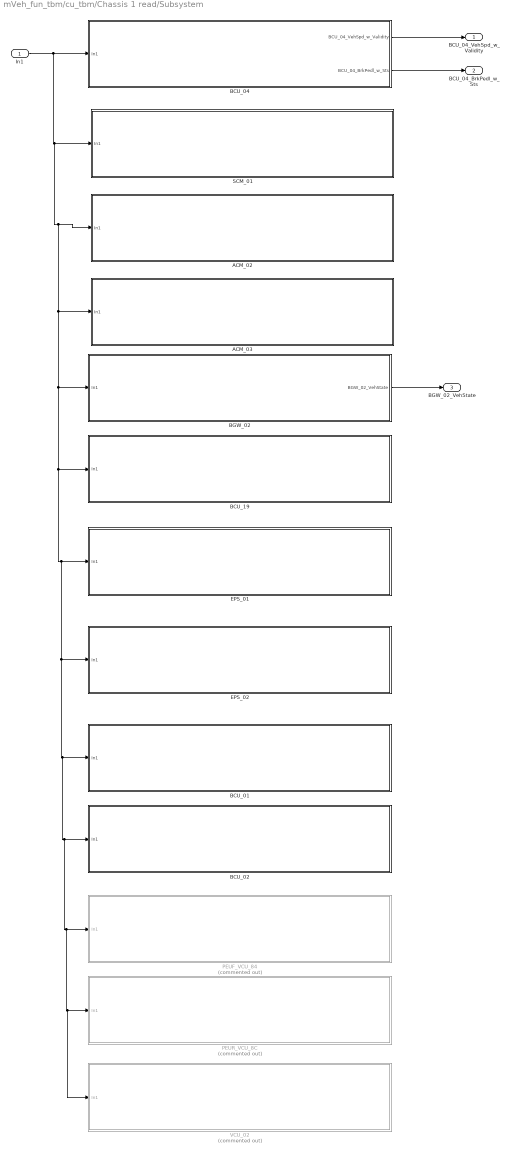
== system mVeh_fun_tbm/cu_tbm/Chassis 1 read/Subsystem ==
  In1 : Inport
  ACM_02 : Subsystem
  ACM_03 : Subsystem
  BCU_01 : Subsystem
  BCU_02 : Subsystem
  BCU_04 : Subsystem
  BCU_19 : Subsystem
  BGW_02 : Subsystem
  EPS_01 : Subsystem
  EPS_02 : Subsystem
  PEUF_VCU_84 : Subsystem  Commented=on
  PEUR_VCU_8C : Subsystem  Commented=on
  SCM_01 : Subsystem
  VCU_02 : Subsystem  Commented=on
  BCU_04_VehSpd_w_Validity : Outport
  BCU_04_BrkPedl_w_Sts : Outport  Port=2
  BGW_02_VehState : Outport  Port=3
  wires:
  BCU_04/1(BCU_04_VehSpd_w_Validity) -> BCU_04_VehSpd_w_Validity/1
  BCU_04/2(BCU_04_BrkPedl_w_Sts) -> BCU_04_BrkPedl_w_Sts/1
  BGW_02/1(BGW_02_VehState) -> BGW_02_VehState/1
  In1/1 -> ACM_03/1(In1), EPS_02/1(In1), VCU_02/1(In1), PEUR_VCU_8C/1(In1), PEUF_VCU_84/1(In1), BCU_02/1(In1), BCU_01/1(In1), EPS_01/1(In1), BCU_19/1(In1), BGW_02/1(In1), ACM_02/1(In1), SCM_01/1(In1), BCU_04/1(In1)

== system mVeh_fun_tbm/cu_tbm/Height Snr/Subsystem ==
  In1 : Inport
  Height Snr : Subsystem
  Height : Outport
  wires:
  In1/1 -> Height Snr/1(In1)
  Height Snr/1(Height) -> Height/1

== system mVeh_fun_tbm/cu_tbm/PVRR read/Subsystem ==
  In1 : Inport
  PVRR : Subsystem
  PVRR_press : Outport
  PVRR_timestamp : Outport  Port=2
  wires:
  In1/1 -> PVRR/1(In1)
  PVRR/1(PVRR_press) -> PVRR_press/1
  PVRR/2(PVRR_timestamp) -> PVRR_timestamp/1

== system mVeh_fun_tbm/cu_tbm/Sensata  Read/Subsystem ==
  In1 : Inport
  TPMS_TireBurst_Matrix : Subsystem
  TPMS_TireBurst : Outport
  wires:
  In1/1 -> TPMS_TireBurst_Matrix/1(In1)
  TPMS_TireBurst_Matrix/1(TPMS_TireBurst*1) -> TPMS_TireBurst/1

== system mVeh_fun_tbm/cu_tbm/Subsystem1/ write TBM_02 ==
  note: TBM_02 10ms
  Input : Inport  PortDimensions=10
  Bus Selector : BusSelector  OutputSignals=LeakActv_spring1,LeakActv_spring2,LeakActv_spring3,LeakActv_spring4,springID,LeakTargPres_spring1,LeakTargPres_spring2,LeakTargPres_spring3,LeakTargPres_spring4,reserved
  CAN Write2 : speedgoatlib_IO691/CAN Write  id=2  ts=0.01  channel=1  messageType=CAN  enableStatusPort=off  canType=CAN (HS)  initValues=[691 2 0.01 0 1 1 0]
  Data Type Conversion{,1..4} (5 alike) : DataTypeConversion  OutDataTypeStr=single  RndMeth=Nearest  SaturateOnIntegerOverflow=off
  Scope : Scope
  Scope2 : Scope  NumInputPorts=8
  TBM_02 : canmsglib/CAN Pack  CANdbFile=.\support\dbc\FCC1_NT2_Chassis1_CAN_Official_Release_V_1_4_DA_01_updated_mod.dbc  MsgList=TBM_02  MsgName=TBM_02  MsgIDType=Standard (11-bit identifier)  MsgIdentifier=128  MsgLength=8  Remote=off  ApplyMinMax=off  BusOutput=off  SignalInfo={'LeakActv_spring1','56','1','BE','unsigned','Standard','0','1','0','0','1';'LeakActv_spring2','57','1','BE','unsigned','Standard','0','1','0','0','1';'LeakActv_spring3','58','1','BE','unsigned','Standard','0','1','0','0','1';'LeakActv_spring4','59','1','BE','unsigned','Standard','0','1','0','0','1';'LeakFirst_springID','60','3','BE','unsigned','Standard','0','1','0','0','7';'LeakTargPres_spring1','17','11','BE','unsigned','Standard','0','1','0','0','2047';'LeakTargPres_spring2','38','11','BE','unsigned','Standard','0','1','0','0','2047';'LeakTargPres_spring3','43','11','BE','unsigned','Standard','0','1','0','0','2047';'LeakTargPres_spring4','48','11','BE','unsigned','Standard','0','1','0','0','2047';'TBM_02_CRC','0','8','BE','unsigned','Standard','0','1','0','0','255';'TBM_02_MsgCntr','12','4','BE','unsigned','Standard','0','1','0','0','15';'TBM_02_reserved','63','1','BE','unsigned','Standard','0','1','0','0','1'}
      settings: DataFormat=CANdb specified signals
  canPack_nt2ch1_v1_4da01_fcc.dbc:TBM_02 : Subsystem
  lib_gen_canMsgCntr : libtb_gen_canMsgCntr/lib_gen_canMsgCntr  SystemSampleTime=-1  VariantActivationTime=update diagram  AllowFlexibleInterface=on  Latency=0  AutoFrameSizeCalculation=off
  pulseGen : DiscretePulseGenerator  PulseType=Time based  Period=0.01  PulseWidth=50
  wires:
  TBM_02/1 -> CAN Write2/1
  pulseGen/1 -> canPack_nt2ch1_v1_4da01_fcc.dbc:TBM_02/Trigger, lib_gen_canMsgCntr/Trigger
  Input/1 -> Bus Selector/1
  Bus Selector/1 -> Data Type Conversion2/1  "<LeakActv_spring1>"
  Bus Selector/2 -> Data Type Conversion1/1  "<LeakActv_spring2>"
  Bus Selector/3 -> Data Type Conversion3/1  "<LeakActv_spring3>"
  Bus Selector/4 -> Data Type Conversion4/1  "<LeakActv_spring4>"
  Bus Selector/5 -> canPack_nt2ch1_v1_4da01_fcc.dbc:TBM_02/5(LeakFirst_springID), TBM_02/5  "<springID>"
  Bus Selector/6 -> Scope2/5, TBM_02/6, canPack_nt2ch1_v1_4da01_fcc.dbc:TBM_02/6(LeakTargPres_spring1)  "<LeakTargPres_spring1>"
  Bus Selector/7 -> Scope2/6, TBM_02/7, canPack_nt2ch1_v1_4da01_fcc.dbc:TBM_02/7(LeakTargPres_spring2)  "<LeakTargPres_spring2>"
  Bus Selector/8 -> Scope2/7, TBM_02/8, canPack_nt2ch1_v1_4da01_fcc.dbc:TBM_02/8(LeakTargPres_spring3)  "<LeakTargPres_spring3>"
  Bus Selector/9 -> Scope2/8, TBM_02/9, canPack_nt2ch1_v1_4da01_fcc.dbc:TBM_02/9(LeakTargPres_spring4)  "<LeakTargPres_spring4>"
  Bus Selector/10 -> TBM_02/12, canPack_nt2ch1_v1_4da01_fcc.dbc:TBM_02/12(TBM_02_reserved)  "<reserved>"
  canPack_nt2ch1_v1_4da01_fcc.dbc:TBM_02/1(crc_8) -> TBM_02/10
  Data Type Conversion/1 -> TBM_02/11, canPack_nt2ch1_v1_4da01_fcc.dbc:TBM_02/11(TBM_02_MsgCntr), Scope/1
  lib_gen_canMsgCntr/1 -> Data Type Conversion/1
  Data Type Conversion1/1 -> Scope2/2, canPack_nt2ch1_v1_4da01_fcc.dbc:TBM_02/2(LeakActv_spring2), TBM_02/2
  Data Type Conversion2/1 -> Scope2/1, canPack_nt2ch1_v1_4da01_fcc.dbc:TBM_02/1(LeakActv_spring1), TBM_02/1
  Data Type Conversion3/1 -> Scope2/3, canPack_nt2ch1_v1_4da01_fcc.dbc:TBM_02/3(LeakActv_spring3), TBM_02/3
  Data Type Conversion4/1 -> Scope2/4, canPack_nt2ch1_v1_4da01_fcc.dbc:TBM_02/4(LeakActv_spring4), TBM_02/4

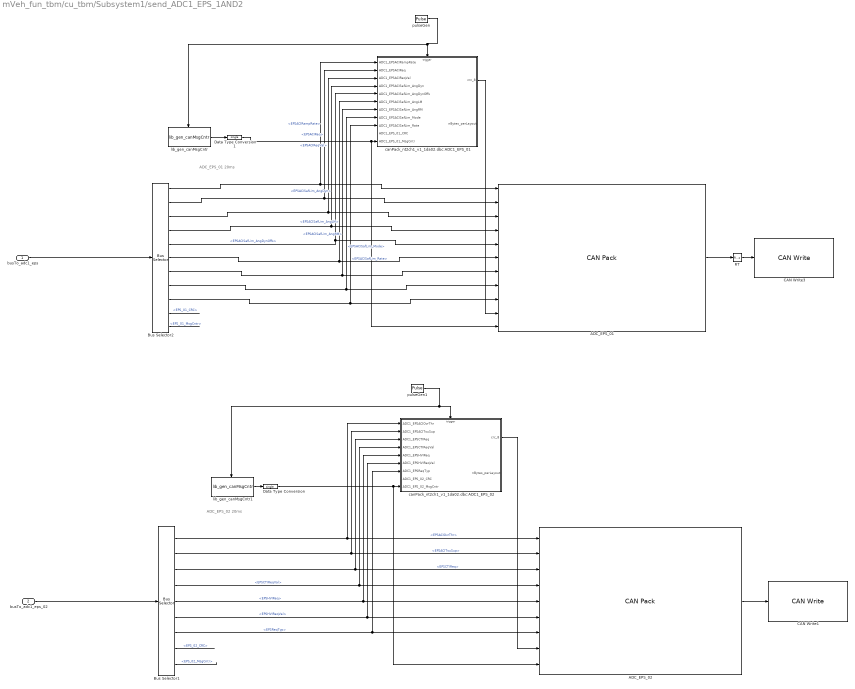
== system mVeh_fun_tbm/cu_tbm/Subsystem1/send_ADC1_EPS_1AND2 ==
  note: ADC_EPS_01 20ms
  note: ADC_EPS_02 20ms
  busTo_adc1_eps : Inport
  busTo_adc1_eps_02 : Inport  Port=2
  ADC_EPS_01 : canmsglib/CAN Pack  CANdbFile=.\support\dbc\NIO_NT2_Chassis1_CAN_Official_Release_V_1_1_DA_02.dbc  MsgList=ADC1_EPS_01  MsgName=ADC1_EPS_01  MsgIDType=Standard (11-bit identifier)  MsgIdentifier=112  MsgLength=8  Remote=off  ApplyMinMax=off  BusOutput=off  SignalInfo={'ADC1_EPSACIRampRate','57','2','BE','unsigned','Standard','0','1','0','0','3';'ADC1_EPSACIReq','41','15','BE','unsigned','Standard','0','0.1','-1638.4','-1638.4','1638.3';'ADC1_EPSACIReqVal','40','1','BE','unsigned','Standard','0','1','0','0','1';'ADC1_EPSACISafLim_AngDyn','25','15','BE','unsigned','Standard','0','0.1','-1638.4','-1638.4','1638.3';'ADC1_EPSACISafLim_AngDynOffs','8','4','BE','unsigned','Standard','0','1','0','0','15';'ADC1_EPSACISafLim_AngLM','52','4','BE','unsigned','Standard','0','1','0','0','15';'ADC1_EPSACISafLim_AngRM','48','4','BE','unsigned','Standard','0','1','0','0','15';'ADC1_EPSACISafLim_Mode','24','1','BE','unsigned','Standard','0','1','0','0','1';'ADC1_EPSACISafLim_Rate','59','5','BE','unsigned','Standard','0','1','0','0','31';'ADC1_EPS_01_CRC','0','8','BE','unsigned','Standard','0','1','0','0','255';'ADC1_EPS_01_MsgCntr','12','4','BE','unsigned','Standard','0','1','0','0','15'}
      settings: DataFormat=CANdb specified signals
  ADC_EPS_02 : canmsglib/CAN Pack  CANdbFile=.\support\dbc\NIO_NT2_Chassis1_CAN_Official_Release_V_1_1_DA_02.dbc  MsgList=ADC1_EPS_02  MsgName=ADC1_EPS_02  MsgIDType=Standard (11-bit identifier)  MsgIdentifier=113  MsgLength=8  Remote=off  ApplyMinMax=off  BusOutput=off  SignalInfo={'ADC1_EPSACIOvrThr','18','3','BE','unsigned','Standard','0','1','0','0','7';'ADC1_EPSACITsuSup','21','3','BE','unsigned','Standard','0','1','0','0','7';'ADC1_EPSCTIReq','24','10','BE','unsigned','Standard','0','0.02','-10.24','-10.24','10.22';'ADC1_EPSCTIReqVal','39','1','BE','unsigned','Standard','0','1','0','0','1';'ADC1_EPSHVIReq','9','3','BE','unsigned','Standard','0','1','0','0','7';'ADC1_EPSHVIReqVal','8','1','BE','unsigned','Standard','0','1','0','0','1';'ADC1_EPSReqTyp','36','3','BE','unsigned','Standard','0','1','0','0','7';'ADC1_EPS_02_CRC','0','8','BE','unsigned','Standard','0','1','0','0','255';'ADC1_EPS_02_MsgCntr','12','4','BE','unsigned','Standard','0','1','0','0','15'}
      settings: DataFormat=CANdb specified signals
  Bus Selector1 : BusSelector  OutputSignals=EPSACIOvrThr,EPSACITsuSup,EPSCTIReq,EPSCTIReqVal,EPSHVIReq,EPSHVIReqVal,EPSReqTyp,EPS_02_CRC,EPS_02_MsgCntr
  Bus Selector2 : BusSelector  OutputSignals=EPSACIRampRate,EPSACIReq,EPSACIReqVal,EPSACISafLim_AngDyn,EPSACISafLim_AngDynOffs,EPSACISafLim_AngLM,EPSACISafLim_AngRM,EPSACISafLim_Mode,EPSACISafLim_Rate,EPS_01_CRC,EPS_01_MsgCntr
  CAN Write1 : speedgoatlib_IO691/CAN Write  id=2  ts=0.02  channel=1  messageType=CAN  enableStatusPort=off  canType=CAN (HS)  initValues=[691 2 0.02 0 1 1 0]
  CAN Write3 : speedgoatlib_IO691/CAN Write  id=2  ts=0.02  channel=1  messageType=CAN  enableStatusPort=off  canType=CAN (HS)  initValues=[691 2 0.02 0 1 1 0]
  Data Type Conversion : DataTypeConversion  OutDataTypeStr=single  RndMeth=Nearest  SaturateOnIntegerOverflow=off
  Data Type Conversion1 : DataTypeConversion  OutDataTypeStr=single  RndMeth=Nearest  SaturateOnIntegerOverflow=off
  RT : RateTransition  OutPortSampleTime=0.02
  canPack_nt2ch1_v1_1da02.dbc:ADC1_EPS_01 : Subsystem
  canPack_nt2ch1_v1_1da02.dbc:ADC1_EPS_02 : Subsystem
  lib_gen_canMsgCntr : libtb_gen_canMsgCntr/lib_gen_canMsgCntr  SystemSampleTime=-1  VariantActivationTime=update diagram  AllowFlexibleInterface=on  Latency=0  AutoFrameSizeCalculation=off
  lib_gen_canMsgCntr1 : libtb_gen_canMsgCntr/lib_gen_canMsgCntr  SystemSampleTime=-1  VariantActivationTime=update diagram  AllowFlexibleInterface=on  Latency=0  AutoFrameSizeCalculation=off
  pulseGen : DiscretePulseGenerator  PulseType=Time based  Period=0.02  PulseWidth=50
  pulseGen1 : DiscretePulseGenerator  PulseType=Time based  Period=0.02  PulseWidth=50
  wires:
  busTo_adc1_eps/1 -> Bus Selector2/1
  Bus Selector1/3 -> canPack_nt2ch1_v1_1da02.dbc:ADC1_EPS_02/3(ADC1_EPSCTIReq), ADC_EPS_02/3  "<EPSCTIReq>"
  Bus Selector1/5 -> canPack_nt2ch1_v1_1da02.dbc:ADC1_EPS_02/5(ADC1_EPSHVIReq), ADC_EPS_02/5  "<EPSHVIReq>"
  Bus Selector1/6 -> canPack_nt2ch1_v1_1da02.dbc:ADC1_EPS_02/6(ADC1_EPSHVIReqVal), ADC_EPS_02/6  "<EPSHVIReqVal>"
  busTo_adc1_eps_02/1 -> Bus Selector1/1
  Bus Selector1/4 -> canPack_nt2ch1_v1_1da02.dbc:ADC1_EPS_02/4(ADC1_EPSCTIReqVal), ADC_EPS_02/4  "<EPSCTIReqVal>"
  Bus Selector1/1 -> canPack_nt2ch1_v1_1da02.dbc:ADC1_EPS_02/1(ADC1_EPSACIOvrThr), ADC_EPS_02/1  "<EPSACIOvrThr>"
  Bus Selector1/2 -> canPack_nt2ch1_v1_1da02.dbc:ADC1_EPS_02/2(ADC1_EPSACITsuSup), ADC_EPS_02/2  "<EPSACITsuSup>"
  Bus Selector2/1 -> canPack_nt2ch1_v1_1da02.dbc:ADC1_EPS_01/1(ADC1_EPSACIRampRate), ADC_EPS_01/1  "<EPSACIRampRate>"
  Bus Selector2/2 -> canPack_nt2ch1_v1_1da02.dbc:ADC1_EPS_01/2(ADC1_EPSACIReq), ADC_EPS_01/2  "<EPSACIReq>"
  Bus Selector2/3 -> canPack_nt2ch1_v1_1da02.dbc:ADC1_EPS_01/3(ADC1_EPSACIReqVal), ADC_EPS_01/3  "<EPSACIReqVal>"
  Bus Selector2/4 -> canPack_nt2ch1_v1_1da02.dbc:ADC1_EPS_01/4(ADC1_EPSACISafLim_AngDyn), ADC_EPS_01/4  "<EPSACISafLim_AngDyn>"
  Bus Selector2/5 -> canPack_nt2ch1_v1_1da02.dbc:ADC1_EPS_01/5(ADC1_EPSACISafLim_AngDynOffs), ADC_EPS_01/5  "<EPSACISafLim_AngDynOffs>"
  Bus Selector2/6 -> canPack_nt2ch1_v1_1da02.dbc:ADC1_EPS_01/6(ADC1_EPSACISafLim_AngLM), ADC_EPS_01/6  "<EPSACISafLim_AngLM>"
  Bus Selector2/7 -> canPack_nt2ch1_v1_1da02.dbc:ADC1_EPS_01/7(ADC1_EPSACISafLim_AngRM), ADC_EPS_01/7  "<EPSACISafLim_AngRM>"
  Bus Selector2/8 -> canPack_nt2ch1_v1_1da02.dbc:ADC1_EPS_01/8(ADC1_EPSACISafLim_Mode), ADC_EPS_01/8  "<EPSACISafLim_Mode>"
  Bus Selector2/9 -> canPack_nt2ch1_v1_1da02.dbc:ADC1_EPS_01/9(ADC1_EPSACISafLim_Rate), ADC_EPS_01/9  "<EPSACISafLim_Rate>"
  canPack_nt2ch1_v1_1da02.dbc:ADC1_EPS_01/1(crc_8) -> ADC_EPS_01/10
  ADC_EPS_01/1 -> RT/1
  ADC_EPS_02/1 -> CAN Write1/1
  Bus Selector1/7 -> canPack_nt2ch1_v1_1da02.dbc:ADC1_EPS_02/7(ADC1_EPSReqTyp), ADC_EPS_02/7  "<EPSReqTyp>"
  pulseGen/1 -> canPack_nt2ch1_v1_1da02.dbc:ADC1_EPS_01/Trigger, lib_gen_canMsgCntr/Trigger
  pulseGen1/1 -> canPack_nt2ch1_v1_1da02.dbc:ADC1_EPS_02/Trigger, lib_gen_canMsgCntr1/Trigger
  Bus Selector2/10 -> ?  "<EPS_01_CRC>"
  Bus Selector2/11 -> ?  "<EPS_01_MsgCntr>"
  Bus Selector1/8 -> ?  "<EPS_02_CRC>"
  Bus Selector1/9 -> ?  "<EPS_02_MsgCntr>"
  lib_gen_canMsgCntr/1 -> Data Type Conversion1/1
  lib_gen_canMsgCntr1/1 -> Data Type Conversion/1
  Data Type Conversion/1 -> canPack_nt2ch1_v1_1da02.dbc:ADC1_EPS_02/9(ADC1_EPS_02_MsgCntr), ADC_EPS_02/9
  Data Type Conversion1/1 -> canPack_nt2ch1_v1_1da02.dbc:ADC1_EPS_01/11(ADC1_EPS_01_MsgCntr), ADC_EPS_01/11
  canPack_nt2ch1_v1_1da02.dbc:ADC1_EPS_02/1(crc_8) -> ADC_EPS_02/8
  RT/1 -> CAN Write3/1
